simulink model "model_lqg_int"  (R2022b)
settings: Solver=VariableStepAuto  StartTime=0.0  StopTime=40.0  RelTol=1e-3
values from neighbouring files (symbols this model uses):
  A = J.A    [DK_iteration.m]    (also in Hinf_controller_hinfsyn.m = Jo.A; Hinf_controller_mixsyn.m = Jo.A; LQG_integrator.m = [J.A Znp;-J.C Zpp]; LQG_with_integrator.m = [J.A Znp;-J.C Zpp])
  B = J.B    [DK_iteration.m]    (also in Hinf_controller_hinfsyn.m = Jo.B; Hinf_controller_mixsyn.m = Jo.B; LQG_integrator.m = [J.B;-J.D]; LQG_with_integrator.m = [J.B;-J.D])
  C = J.C    [DK_iteration.m]    (also in Hinf_controller_hinfsyn.m = Jo.C; Hinf_controller_mixsyn.m = Jo.C; LQG_integrator.m = [J.C Zpp]; LQG_with_integrator.m = [J.C Zpp])
  J = get_linearization()    [DK_iteration.m]    (also in LQG.m; LQG_integrator.m; LQG_with_integrator.m; mu_analysis.m = get_linearization_lqg())
  Kr = lqr(J.A,J.B,Q,R)    [LQG.m]    (also in LQG_integrator.m = lqr(A,B,Q,R); LQG_with_integrator.m = lqr(A,B,Q,R))
undefined symbols (not defined in the file or in its folder): Ke, std_dev_dx, std_dev_dy, std_dev_phi_dot, std_dev_psi, X_start_int
libraries: simulink x1
settings Model: Creator=alexi  LastModifiedBy=franc

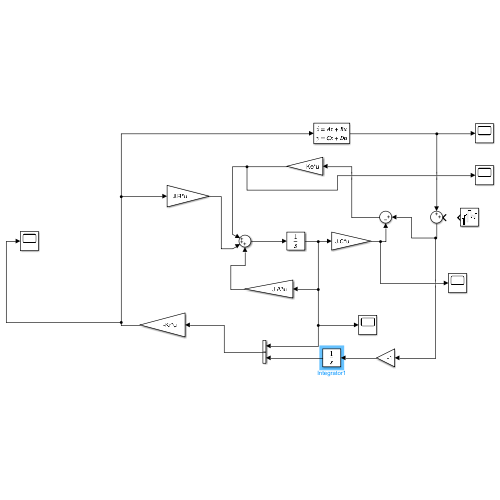
[thumbnail: Simulink's stored preview of the top-level diagram]
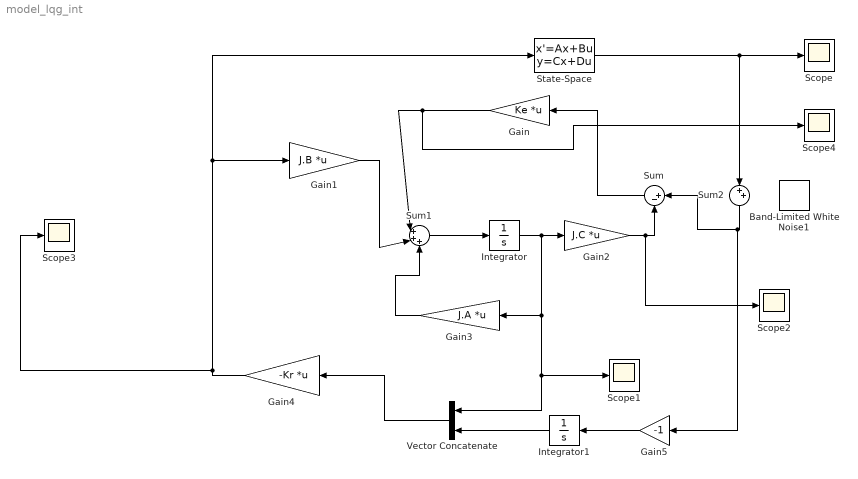
== system model_lqg_int ==
  Band-Limited White Noise1 : simulink/Sources/Band-Limited White Noise  Cov=[std_dev_dx; std_dev_dy; std_dev_phi_dot; std_dev_psi]  Ts=0.1  seed=[23341]
  Gain : Gain  Gain=Ke  Multiplication=Matrix(K*u)
  Gain1 : Gain  Gain=J.B  Multiplication=Matrix(K*u)
  Gain2 : Gain  Gain=J.C  Multiplication=Matrix(K*u)
  Gain3 : Gain  Gain=J.A  Multiplication=Matrix(K*u)
  Gain4 : Gain  Gain=-Kr  Multiplication=Matrix(K*u)
  Gain5 : Gain  Gain=-1
  Integrator : Integrator
  Integrator1 : Integrator
  Scope{,1..4} (5 alike) : Scope
  State-Space : StateSpace  A=A  B=B  C=C  D=J.D  InitialCondition=X_start_int
  Sum : Sum  Inputs=|+-
  Sum1 : Sum  Inputs=|+++
  Sum2 : Sum  Inputs=|++
  Vector Concatenate : Concatenate
  wires:
  State-Space/1 -> Scope/1, Sum2/1
  Sum1/1 -> Integrator/1
  Gain1/1 -> Sum1/2
  Sum/1 -> Gain/1
  Gain3/1 -> Sum1/3
  Sum2/1 -> Gain5/1, Sum/1
  Integrator/1 -> Vector Concatenate/1, Scope1/1, Gain3/1, Gain2/1
  Gain/1 -> Scope4/1, Sum1/1
  Gain2/1 -> Scope2/1, Sum/2
  Gain4/1 -> Scope3/1, State-Space/1, Gain1/1
  Gain5/1 -> Integrator1/1
  Vector Concatenate/1 -> Gain4/1
  Integrator1/1 -> Vector Concatenate/2
